simulink model "Simscape_Actuated_Robot"  (R2025b)
settings: Solver=ode45  StartTime=0.0  StopTime=20  RelTol=1e-3
InitFcn:
  | run("init.m");
values from neighbouring files (symbols this model uses):
  q0_guess = [pi/3; -pi/6; pi/3]    [init.m]
  q_init = [pi/6,-pi/3, 0,pi/6,-pi/3,0]    [init.m]
  Ts = 1e-3    (= 0.001)    [init.m]
undefined symbols (not defined in the file or in its folder): robot_params, X, Y, Z
libraries: sm_lib x48, nesl_utility x48
(part 2 of 3)

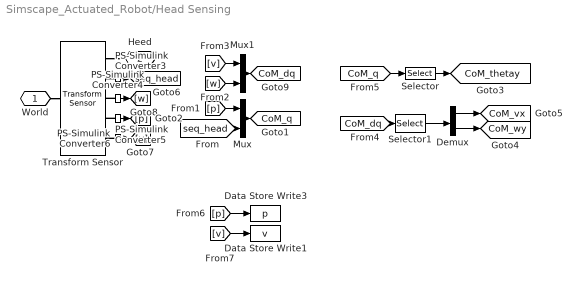
== system Simscape_Actuated_Robot/Head Sensing ==
  Data Store Write1 : DataStoreWrite  DataStoreName=v  DataStoreElements=v  EnableIndexing=on  NumberOfDimensions=2  IndexOptions=Index vector (dialog),Index vector (dialog)  Indices=[1 2 3],[2]  OutputSizes=1,1
  Data Store Write3 : DataStoreWrite  DataStoreName=p  DataStoreElements=p  EnableIndexing=on  NumberOfDimensions=2  IndexOptions=Index vector (dialog),Index vector (dialog)  Indices=[1 2 3],[1]  OutputSizes=1,1
  Demux : Demux  Outputs=2
  Mux : Mux  Inputs=2
  Mux1 : Mux  Inputs=2
  PS-Simulink Converter{3..6} (4 alike) : nesl_utility/PS-Simulink Converter  PhysicalDomain=network_engine_domain  SubClassName=ps_output  LeftPortType=input  RightPortType=output  PseudoPeriodic=off  Frequencies=[]  VectorFormat=inherit  Unit=inherit  AffineConversion=off
  Selector : Selector  InputPortWidth=6  IndexOptions=Index vector (dialog)  Indices=5  OutputSizes=1
  Selector1 : Selector  InputPortWidth=6  IndexOptions=Index vector (dialog)  Indices=[1 5]  OutputSizes=1
  Transform Sensor : sm_lib/Frames and Transforms/Transform Sensor  MeasurementFrame=World  RotationSequence=XYZ  SenseAngle=off  SenseAxis=off  SenseQ=off  SenseR=off  SenseRotationSequence=on  SenseOmegaX=off  SenseOmegaY=off  SenseOmegaZ=off  SenseOmega=on  SenseQDot=off  SenseRDot=off  SenseRotationSequenceDot=off  SenseAlphaX=off  SenseAlphaY=off  SenseAlphaZ=off  SenseAlpha=off  SenseQDDot=off  SenseRDDot=off  SenseX=off  SenseY=off  SenseZ=off  SenseXYZ=on  SenseRad=off  SenseAzim=off  SenseDist=off  SenseInc=off  SenseXDot=off  SenseYDot=off  SenseZDot=off  SenseXYZDot=on  SenseRadDot=off  SenseAzimDot=off  SenseDistDot=off  SenseIncDot=off  SenseXDDot=off  SenseYDDot=off  SenseZDDot=off  SenseXYZDDot=off  SenseRadDDot=off  SenseAzimDDot=off  SenseDistDDot=off  SenseIncDDot=off
  World : PMIOPort  Side=Right
  Heed : PMIOPort  Port=2  Side=Left
  tag scope: CoM_dq=global, CoM_q=global, CoM_thetay=global, CoM_vx=global, CoM_wy=global, seq_head=global
  wires:
  Selector/1 -> [CoM_thetay]
  PS-Simulink Converter5/1 -> [p]
  PS-Simulink Converter3/1 -> [seq_head]
  [p] -> Mux/1
  [seq_head] -> Mux/2
  PS-Simulink Converter6/1 -> [v]
  PS-Simulink Converter4/1 -> [w]
  Mux/1 -> [CoM_q]
  Mux1/1 -> [CoM_dq]
  [w] -> Mux1/2
  [v] -> Mux1/1
  [CoM_dq] -> Selector1/1
  Selector1/1 -> Demux/1
  Demux/1 -> [CoM_vx]
  Demux/2 -> [CoM_wy]
  [CoM_q] -> Selector/1
  [p] -> Data Store Write3/1
  [v] -> Data Store Write1/1
  connections:
  PS-Simulink Converter6/LConn1 -- Transform Sensor/RConn5
  PS-Simulink Converter5/LConn1 -- Transform Sensor/RConn4
  PS-Simulink Converter4/LConn1 -- Transform Sensor/RConn3
  Transform Sensor/RConn2 -- PS-Simulink Converter3/LConn1
  Transform Sensor/RConn1 -- Heed/RConn1
  World/RConn1 -- Transform Sensor/LConn1

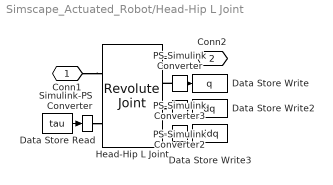
== system Simscape_Actuated_Robot/Head-Hip L Joint  ==
  Data Store Read : DataStoreRead  DataStoreName=tau  DataStoreElements=tau  EnableIndexing=on  IndexOptions=Index vector (dialog)  Indices=4  OutputSizes=1
  Data Store Write : DataStoreWrite  DataStoreName=q  DataStoreElements=q  EnableIndexing=on  IndexOptions=Index vector (dialog)  Indices=4  OutputSizes=1
  Data Store Write2 : DataStoreWrite  DataStoreName=dq  DataStoreElements=dq  EnableIndexing=on  IndexOptions=Index vector (dialog)  Indices=4  OutputSizes=1
  Data Store Write3 : DataStoreWrite  DataStoreName=ddq  DataStoreElements=ddq  EnableIndexing=on  IndexOptions=Index vector (dialog)  Indices=4  OutputSizes=1
  "Head-Hip L Joint " : sm_lib/Joints/Revolute Joint  JointMode=Normal  CompositeWrenchDir=FollowerOnBase  CompositeWrenchFrame=BaseFrame  SenseConstraintForce=off  SenseConstraintTorque=off  SenseTotalForce=off  SenseTotalTorque=off  PositionTargetSpecify=on  PositionTargetPriority=High  PositionTargetValue=q_init(4)  PositionTargetValueUnits=rad  VelocityTargetSpecify=off  VelocityTargetPriority=High  VelocityTargetValue=0  VelocityTargetValueUnits=rad/s  EquilibriumPosition=0  EquilibriumPositionUnits=rad  SpringStiffness=Motor_stiffness  SpringStiffnessUnits=N*m/deg  DampingCoefficient=Motor_damping  DampingCoefficientUnits=N*m/(deg/s)  LowerLimitSpecify=off  LowerLimitBound=-90  LowerLimitBoundUnits=deg  LowerLimitStiffness=1e4  LowerLimitStiffnessUnits=N*m/deg  LowerLimitDamping=10  LowerLimitDampingUnits=N*m/(deg/s)  LowerLimitTransitionRegionWidth=0.1  LowerLimitTransitionRegionWidthUnits=deg  UpperLimitSpecify=off  UpperLimitBound=90  UpperLimitBoundUnits=deg  UpperLimitStiffness=1e4  UpperLimitStiffnessUnits=N*m/deg  UpperLimitDamping=10  UpperLimitDampingUnits=N*m/(deg/s)  UpperLimitTransitionRegionWidth=0.1  UpperLimitTransitionRegionWidthUnits=deg  TorqueActuationMode=InputTorque  MotionActuationMode=ComputedMotion  SensePosition=on  SenseVelocity=on  SenseAcceleration=on  SenseTorqueForce=off  SenseLowerLimitTorqueForce=off  SenseUpperLimitTorqueForce=off
  PS-Simulink Converter : nesl_utility/PS-Simulink Converter  PhysicalDomain=network_engine_domain  SubClassName=ps_output  LeftPortType=input  RightPortType=output  PseudoPeriodic=off  Frequencies=[]  VectorFormat=1-D array  Unit=rad  AffineConversion=off
  PS-Simulink Converter2 : nesl_utility/PS-Simulink Converter  PhysicalDomain=network_engine_domain  SubClassName=ps_output  LeftPortType=input  RightPortType=output  PseudoPeriodic=off  Frequencies=[]  VectorFormat=1-D array  Unit=rad/s  AffineConversion=off
  PS-Simulink Converter3 : nesl_utility/PS-Simulink Converter  PhysicalDomain=network_engine_domain  SubClassName=ps_output  LeftPortType=input  RightPortType=output  PseudoPeriodic=off  Frequencies=[]  VectorFormat=inherit  Unit=inherit  AffineConversion=off
  Simulink-PS Converter : nesl_utility/Simulink-PS Converter  PhysicalDomain=network_engine_domain  SubClassName=ps_input  LeftPortType=input  RightPortType=output  PseudoPeriodic=off  Frequencies=[]  NoiseDistribution=none  NoiseParameters=[]  Unit=N*m  AffineConversion=off  FilteringAndDerivatives=provide  SimscapeFilterOrder=1  InputFilterTimeConstant=0.001  UdotUserProvided=0
  Conn1 : PMIOPort  Side=Left
  Conn2 : PMIOPort  Port=2  Side=Right
  wires:
  PS-Simulink Converter/1 -> Data Store Write/1
  PS-Simulink Converter2/1 -> Data Store Write2/1
  PS-Simulink Converter3/1 -> Data Store Write3/1
  Data Store Read/1 -> Simulink-PS Converter/1
  connections:
  Conn2/RConn1 -- "Head-Hip L Joint "/RConn1
  Conn1/RConn1 -- "Head-Hip L Joint "/LConn1
  PS-Simulink Converter/LConn1 -- "Head-Hip L Joint "/RConn2
  "Head-Hip L Joint "/RConn3 -- PS-Simulink Converter2/LConn1
  "Head-Hip L Joint "/RConn4 -- PS-Simulink Converter3/LConn1
  Simulink-PS Converter/RConn1 -- "Head-Hip L Joint "/LConn2

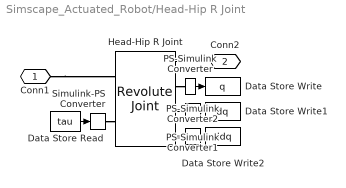
== system Simscape_Actuated_Robot/Head-Hip R Joint  ==
  Data Store Read : DataStoreRead  DataStoreName=tau  DataStoreElements=tau  EnableIndexing=on  IndexOptions=Index vector (dialog)  Indices=1  OutputSizes=1
  Data Store Write : DataStoreWrite  DataStoreName=q  DataStoreElements=q  EnableIndexing=on  IndexOptions=Index vector (dialog)  Indices=1  OutputSizes=1
  Data Store Write1 : DataStoreWrite  DataStoreName=dq  DataStoreElements=dq  EnableIndexing=on  IndexOptions=Index vector (dialog)  Indices=1  OutputSizes=1
  Data Store Write2 : DataStoreWrite  DataStoreName=ddq  DataStoreElements=ddq  EnableIndexing=on  IndexOptions=Index vector (dialog)  Indices=1  OutputSizes=1
  "Head-Hip R Joint " : sm_lib/Joints/Revolute Joint  JointMode=Normal  CompositeWrenchDir=FollowerOnBase  CompositeWrenchFrame=BaseFrame  SenseConstraintForce=off  SenseConstraintTorque=off  SenseTotalForce=off  SenseTotalTorque=off  PositionTargetSpecify=on  PositionTargetPriority=High  PositionTargetValue=q_init(1)  PositionTargetValueUnits=rad  VelocityTargetSpecify=off  VelocityTargetPriority=High  VelocityTargetValue=0  VelocityTargetValueUnits=deg/s  EquilibriumPosition=0  EquilibriumPositionUnits=rad  SpringStiffness=Motor_stiffness  SpringStiffnessUnits=N*m/deg  DampingCoefficient=Motor_damping  DampingCoefficientUnits=N*m/(deg/s)  LowerLimitSpecify=off  LowerLimitBound=-90  LowerLimitBoundUnits=deg  LowerLimitStiffness=1e4  LowerLimitStiffnessUnits=N*m/deg  LowerLimitDamping=10  LowerLimitDampingUnits=N*m/(deg/s)  LowerLimitTransitionRegionWidth=0.1  LowerLimitTransitionRegionWidthUnits=deg  UpperLimitSpecify=off  UpperLimitBound=90  UpperLimitBoundUnits=deg  UpperLimitStiffness=1e4  UpperLimitStiffnessUnits=N*m/deg  UpperLimitDamping=10  UpperLimitDampingUnits=N*m/(deg/s)  UpperLimitTransitionRegionWidth=0.1  UpperLimitTransitionRegionWidthUnits=deg  TorqueActuationMode=InputTorque  MotionActuationMode=ComputedMotion  SensePosition=on  SenseVelocity=on  SenseAcceleration=on  SenseTorqueForce=off  SenseLowerLimitTorqueForce=off  SenseUpperLimitTorqueForce=off
  PS-Simulink Converter : nesl_utility/PS-Simulink Converter  PhysicalDomain=network_engine_domain  SubClassName=ps_output  LeftPortType=input  RightPortType=output  PseudoPeriodic=off  Frequencies=[]  VectorFormat=1-D array  Unit=rad  AffineConversion=off
  PS-Simulink Converter1 : nesl_utility/PS-Simulink Converter  PhysicalDomain=network_engine_domain  SubClassName=ps_output  LeftPortType=input  RightPortType=output  PseudoPeriodic=off  Frequencies=[]  VectorFormat=1-D array  Unit=rad/s  AffineConversion=off
  PS-Simulink Converter2 : nesl_utility/PS-Simulink Converter  PhysicalDomain=network_engine_domain  SubClassName=ps_output  LeftPortType=input  RightPortType=output  PseudoPeriodic=off  Frequencies=[]  VectorFormat=1-D array  Unit=inherit  AffineConversion=off
  Simulink-PS Converter : nesl_utility/Simulink-PS Converter  PhysicalDomain=network_engine_domain  SubClassName=ps_input  LeftPortType=input  RightPortType=output  PseudoPeriodic=off  Frequencies=[]  NoiseDistribution=none  NoiseParameters=[]  Unit=N*m  AffineConversion=off  FilteringAndDerivatives=provide  SimscapeFilterOrder=1  InputFilterTimeConstant=0.001  UdotUserProvided=0
  Conn1 : PMIOPort  Side=Left
  Conn2 : PMIOPort  Port=2  Side=Right
  wires:
  PS-Simulink Converter/1 -> Data Store Write/1
  PS-Simulink Converter1/1 -> Data Store Write1/1
  PS-Simulink Converter2/1 -> Data Store Write2/1
  Data Store Read/1 -> Simulink-PS Converter/1
  connections:
  PS-Simulink Converter1/LConn1 -- "Head-Hip R Joint "/RConn3
  Conn2/RConn1 -- "Head-Hip R Joint "/RConn1
  "Head-Hip R Joint "/RConn2 -- PS-Simulink Converter/LConn1
  Conn1/RConn1 -- "Head-Hip R Joint "/LConn1
  PS-Simulink Converter2/LConn1 -- "Head-Hip R Joint "/RConn4
  Simulink-PS Converter/RConn1 -- "Head-Hip R Joint "/LConn2

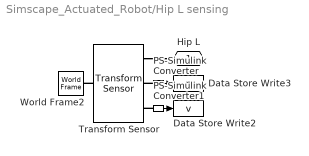
== system Simscape_Actuated_Robot/Hip L sensing ==
  Data Store Write2 : DataStoreWrite  DataStoreName=v  DataStoreElements=v  EnableIndexing=on  NumberOfDimensions=2  IndexOptions=Index vector (dialog),Index vector (dialog)  Indices=[1 2 3],[4]  OutputSizes=1,1
  Data Store Write3 : DataStoreWrite  DataStoreName=p  DataStoreElements=p  EnableIndexing=on  NumberOfDimensions=2  IndexOptions=Index vector (dialog),Index vector (dialog)  Indices=[1 2 3],[4]  OutputSizes=1,1
  PS-Simulink Converter : nesl_utility/PS-Simulink Converter  PhysicalDomain=network_engine_domain  SubClassName=ps_output  LeftPortType=input  RightPortType=output  PseudoPeriodic=off  Frequencies=[]  VectorFormat=inherit  Unit=inherit  AffineConversion=off
  PS-Simulink Converter1 : nesl_utility/PS-Simulink Converter  PhysicalDomain=network_engine_domain  SubClassName=ps_output  LeftPortType=input  RightPortType=output  PseudoPeriodic=off  Frequencies=[]  VectorFormat=inherit  Unit=inherit  AffineConversion=off
  Transform Sensor : sm_lib/Frames and Transforms/Transform Sensor  MeasurementFrame=World  RotationSequence=XYX  SenseAngle=off  SenseAxis=off  SenseQ=off  SenseR=off  SenseRotationSequence=off  SenseOmegaX=off  SenseOmegaY=off  SenseOmegaZ=off  SenseOmega=off  SenseQDot=off  SenseRDot=off  SenseRotationSequenceDot=off  SenseAlphaX=off  SenseAlphaY=off  SenseAlphaZ=off  SenseAlpha=off  SenseQDDot=off  SenseRDDot=off  SenseX=off  SenseY=off  SenseZ=off  SenseXYZ=on  SenseRad=off  SenseAzim=off  SenseDist=off  SenseInc=off  SenseXDot=off  SenseYDot=off  SenseZDot=off  SenseXYZDot=on  SenseRadDot=off  SenseAzimDot=off  SenseDistDot=off  SenseIncDot=off  SenseXDDot=off  SenseYDDot=off  SenseZDDot=off  SenseXYZDDot=off  SenseRadDDot=off  SenseAzimDDot=off  SenseDistDDot=off  SenseIncDDot=off
  World Frame2 : sm_lib/Frames and Transforms/World Frame
  Hip L : PMIOPort  Side=Right
  wires:
  PS-Simulink Converter/1 -> Data Store Write3/1
  PS-Simulink Converter1/1 -> Data Store Write2/1
  connections:
  PS-Simulink Converter/LConn1 -- Transform Sensor/RConn2
  Transform Sensor/RConn1 -- Hip L/RConn1
  Transform Sensor/LConn1 -- World Frame2/RConn1
  PS-Simulink Converter1/LConn1 -- Transform Sensor/RConn3

== system Simscape_Actuated_Robot/Hip R sensing ==
  Data Store Write1 : DataStoreWrite  DataStoreName=v  DataStoreElements=v  EnableIndexing=on  NumberOfDimensions=2  IndexOptions=Index vector (dialog),Index vector (dialog)  Indices=[1 2 3],[2]  OutputSizes=1,1
  Data Store Write3 : DataStoreWrite  DataStoreName=p  DataStoreElements=p  EnableIndexing=on  NumberOfDimensions=2  IndexOptions=Index vector (dialog),Index vector (dialog)  Indices=[1 2 3],[2]  OutputSizes=1,1
  PS-Simulink Converter : nesl_utility/PS-Simulink Converter  PhysicalDomain=network_engine_domain  SubClassName=ps_output  LeftPortType=input  RightPortType=output  PseudoPeriodic=off  Frequencies=[]  VectorFormat=inherit  Unit=inherit  AffineConversion=off
  PS-Simulink Converter1 : nesl_utility/PS-Simulink Converter  PhysicalDomain=network_engine_domain  SubClassName=ps_output  LeftPortType=input  RightPortType=output  PseudoPeriodic=off  Frequencies=[]  VectorFormat=inherit  Unit=inherit  AffineConversion=off
  Transform Sensor : sm_lib/Frames and Transforms/Transform Sensor  MeasurementFrame=World  RotationSequence=XYX  SenseAngle=off  SenseAxis=off  SenseQ=off  SenseR=off  SenseRotationSequence=off  SenseOmegaX=off  SenseOmegaY=off  SenseOmegaZ=off  SenseOmega=off  SenseQDot=off  SenseRDot=off  SenseRotationSequenceDot=off  SenseAlphaX=off  SenseAlphaY=off  SenseAlphaZ=off  SenseAlpha=off  SenseQDDot=off  SenseRDDot=off  SenseX=off  SenseY=off  SenseZ=off  SenseXYZ=on  SenseRad=off  SenseAzim=off  SenseDist=off  SenseInc=off  SenseXDot=off  SenseYDot=off  SenseZDot=off  SenseXYZDot=on  SenseRadDot=off  SenseAzimDot=off  SenseDistDot=off  SenseIncDot=off  SenseXDDot=off  SenseYDDot=off  SenseZDDot=off  SenseXYZDDot=off  SenseRadDDot=off  SenseAzimDDot=off  SenseDistDDot=off  SenseIncDDot=off
  World Frame2 : sm_lib/Frames and Transforms/World Frame
  Hip R : PMIOPort  Side=Right
  wires:
  PS-Simulink Converter/1 -> Data Store Write3/1
  PS-Simulink Converter1/1 -> Data Store Write1/1
  connections:
  Transform Sensor/LConn1 -- World Frame2/RConn1
  Transform Sensor/RConn1 -- Hip R/RConn1
  PS-Simulink Converter/LConn1 -- Transform Sensor/RConn2
  PS-Simulink Converter1/LConn1 -- Transform Sensor/RConn3

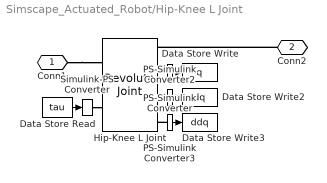
== system Simscape_Actuated_Robot/Hip-Knee L Joint ==
  Data Store Read : DataStoreRead  DataStoreName=tau  DataStoreElements=tau  EnableIndexing=on  IndexOptions=Index vector (dialog)  Indices=5  OutputSizes=1
  Data Store Write : DataStoreWrite  DataStoreName=q  DataStoreElements=q  EnableIndexing=on  IndexOptions=Index vector (dialog)  Indices=5  OutputSizes=1
  Data Store Write2 : DataStoreWrite  DataStoreName=dq  DataStoreElements=dq  EnableIndexing=on  IndexOptions=Index vector (dialog)  Indices=5  OutputSizes=1
  Data Store Write3 : DataStoreWrite  DataStoreName=ddq  DataStoreElements=ddq  EnableIndexing=on  IndexOptions=Index vector (dialog)  Indices=5  OutputSizes=1
  Hip-Knee L Joint : sm_lib/Joints/Revolute Joint  JointMode=Normal  CompositeWrenchDir=FollowerOnBase  CompositeWrenchFrame=BaseFrame  SenseConstraintForce=off  SenseConstraintTorque=off  SenseTotalForce=off  SenseTotalTorque=off  PositionTargetSpecify=on  PositionTargetPriority=High  PositionTargetValue=q_init(5)  PositionTargetValueUnits=rad  VelocityTargetSpecify=off  VelocityTargetPriority=High  VelocityTargetValue=0  VelocityTargetValueUnits=deg/s  EquilibriumPosition=0  EquilibriumPositionUnits=deg  SpringStiffness=Motor_stiffness  SpringStiffnessUnits=N*m/deg  DampingCoefficient=Motor_damping  DampingCoefficientUnits=N*m/(deg/s)  LowerLimitSpecify=off  LowerLimitBound=-90  LowerLimitBoundUnits=deg  LowerLimitStiffness=1e4  LowerLimitStiffnessUnits=N*m/deg  LowerLimitDamping=10  LowerLimitDampingUnits=N*m/(deg/s)  LowerLimitTransitionRegionWidth=0.1  LowerLimitTransitionRegionWidthUnits=deg  UpperLimitSpecify=off  UpperLimitBound=90  UpperLimitBoundUnits=deg  UpperLimitStiffness=1e4  UpperLimitStiffnessUnits=N*m/deg  UpperLimitDamping=10  UpperLimitDampingUnits=N*m/(deg/s)  UpperLimitTransitionRegionWidth=0.1  UpperLimitTransitionRegionWidthUnits=deg  TorqueActuationMode=InputTorque  MotionActuationMode=ComputedMotion  SensePosition=on  SenseVelocity=on  SenseAcceleration=on  SenseTorqueForce=off  SenseLowerLimitTorqueForce=off  SenseUpperLimitTorqueForce=off
  PS-Simulink Converter : nesl_utility/PS-Simulink Converter  PhysicalDomain=network_engine_domain  SubClassName=ps_output  LeftPortType=input  RightPortType=output  PseudoPeriodic=off  Frequencies=[]  VectorFormat=1-D array  Unit=rad  AffineConversion=off
  PS-Simulink Converter2 : nesl_utility/PS-Simulink Converter  PhysicalDomain=network_engine_domain  SubClassName=ps_output  LeftPortType=input  RightPortType=output  PseudoPeriodic=off  Frequencies=[]  VectorFormat=1-D array  Unit=rad/s  AffineConversion=off
  PS-Simulink Converter3 : nesl_utility/PS-Simulink Converter  PhysicalDomain=network_engine_domain  SubClassName=ps_output  LeftPortType=input  RightPortType=output  PseudoPeriodic=off  Frequencies=[]  VectorFormat=inherit  Unit=inherit  AffineConversion=off
  Simulink-PS Converter : nesl_utility/Simulink-PS Converter  PhysicalDomain=network_engine_domain  SubClassName=ps_input  LeftPortType=input  RightPortType=output  PseudoPeriodic=off  Frequencies=[]  NoiseDistribution=none  NoiseParameters=[]  Unit=N*m  AffineConversion=off  FilteringAndDerivatives=provide  SimscapeFilterOrder=1  InputFilterTimeConstant=0.001  UdotUserProvided=0
  Conn1 : PMIOPort  Side=Left
  Conn2 : PMIOPort  Port=2  Side=Right
  wires:
  PS-Simulink Converter/1 -> Data Store Write/1
  PS-Simulink Converter3/1 -> Data Store Write3/1
  PS-Simulink Converter2/1 -> Data Store Write2/1
  Data Store Read/1 -> Simulink-PS Converter/1
  connections:
  Conn2/RConn1 -- Hip-Knee L Joint/RConn1
  Conn1/RConn1 -- Hip-Knee L Joint/LConn1
  PS-Simulink Converter/LConn1 -- Hip-Knee L Joint/RConn2
  PS-Simulink Converter3/LConn1 -- Hip-Knee L Joint/RConn4
  PS-Simulink Converter2/LConn1 -- Hip-Knee L Joint/RConn3
  Simulink-PS Converter/RConn1 -- Hip-Knee L Joint/LConn2

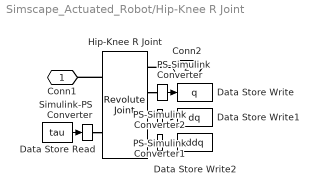
== system Simscape_Actuated_Robot/Hip-Knee R Joint ==
  Data Store Read : DataStoreRead  DataStoreName=tau  DataStoreElements=tau  EnableIndexing=on  IndexOptions=Index vector (dialog)  Indices=2  OutputSizes=1
  Data Store Write : DataStoreWrite  DataStoreName=q  DataStoreElements=q  EnableIndexing=on  IndexOptions=Index vector (dialog)  Indices=2  OutputSizes=1
  Data Store Write1 : DataStoreWrite  DataStoreName=dq  DataStoreElements=dq  EnableIndexing=on  IndexOptions=Index vector (dialog)  Indices=2  OutputSizes=1
  Data Store Write2 : DataStoreWrite  DataStoreName=ddq  DataStoreElements=ddq  EnableIndexing=on  IndexOptions=Index vector (dialog)  Indices=2  OutputSizes=1
  Hip-Knee R Joint : sm_lib/Joints/Revolute Joint  JointMode=Normal  CompositeWrenchDir=FollowerOnBase  CompositeWrenchFrame=BaseFrame  SenseConstraintForce=off  SenseConstraintTorque=off  SenseTotalForce=off  SenseTotalTorque=off  PositionTargetSpecify=on  PositionTargetPriority=High  PositionTargetValue=q_init(2)  PositionTargetValueUnits=rad  VelocityTargetSpecify=off  VelocityTargetPriority=High  VelocityTargetValue=0  VelocityTargetValueUnits=deg/s  EquilibriumPosition=0  EquilibriumPositionUnits=deg  SpringStiffness=Motor_stiffness  SpringStiffnessUnits=N*m/deg  DampingCoefficient=Motor_damping  DampingCoefficientUnits=N*m/(deg/s)  LowerLimitSpecify=off  LowerLimitBound=-90  LowerLimitBoundUnits=deg  LowerLimitStiffness=1e4  LowerLimitStiffnessUnits=N*m/deg  LowerLimitDamping=10  LowerLimitDampingUnits=N*m/(deg/s)  LowerLimitTransitionRegionWidth=0.1  LowerLimitTransitionRegionWidthUnits=deg  UpperLimitSpecify=off  UpperLimitBound=90  UpperLimitBoundUnits=deg  UpperLimitStiffness=1e4  UpperLimitStiffnessUnits=N*m/deg  UpperLimitDamping=10  UpperLimitDampingUnits=N*m/(deg/s)  UpperLimitTransitionRegionWidth=0.1  UpperLimitTransitionRegionWidthUnits=deg  TorqueActuationMode=InputTorque  MotionActuationMode=ComputedMotion  SensePosition=on  SenseVelocity=on  SenseAcceleration=on  SenseTorqueForce=off  SenseLowerLimitTorqueForce=off  SenseUpperLimitTorqueForce=off
  PS-Simulink Converter : nesl_utility/PS-Simulink Converter  PhysicalDomain=network_engine_domain  SubClassName=ps_output  LeftPortType=input  RightPortType=output  PseudoPeriodic=off  Frequencies=[]  VectorFormat=1-D array  Unit=rad  AffineConversion=off
  PS-Simulink Converter1 : nesl_utility/PS-Simulink Converter  PhysicalDomain=network_engine_domain  SubClassName=ps_output  LeftPortType=input  RightPortType=output  PseudoPeriodic=off  Frequencies=[]  VectorFormat=1-D array  Unit=rad/s  AffineConversion=off
  PS-Simulink Converter2 : nesl_utility/PS-Simulink Converter  PhysicalDomain=network_engine_domain  SubClassName=ps_output  LeftPortType=input  RightPortType=output  PseudoPeriodic=off  Frequencies=[]  VectorFormat=inherit  Unit=inherit  AffineConversion=off
  Simulink-PS Converter : nesl_utility/Simulink-PS Converter  PhysicalDomain=network_engine_domain  SubClassName=ps_input  LeftPortType=input  RightPortType=output  PseudoPeriodic=off  Frequencies=[]  NoiseDistribution=none  NoiseParameters=[]  Unit=N*m  AffineConversion=off  FilteringAndDerivatives=provide  SimscapeFilterOrder=1  InputFilterTimeConstant=0.001  UdotUserProvided=0
  Conn1 : PMIOPort  Side=Left
  Conn2 : PMIOPort  Port=2  Side=Right
  wires:
  PS-Simulink Converter/1 -> Data Store Write/1
  PS-Simulink Converter2/1 -> Data Store Write2/1
  PS-Simulink Converter1/1 -> Data Store Write1/1
  Data Store Read/1 -> Simulink-PS Converter/1
  connections:
  Conn2/RConn1 -- Hip-Knee R Joint/RConn1
  Hip-Knee R Joint/LConn1 -- Conn1/RConn1
  Hip-Knee R Joint/RConn2 -- PS-Simulink Converter/LConn1
  PS-Simulink Converter1/LConn1 -- Hip-Knee R Joint/RConn3
  PS-Simulink Converter2/LConn1 -- Hip-Knee R Joint/RConn4
  Simulink-PS Converter/RConn1 -- Hip-Knee R Joint/LConn2

== system Simscape_Actuated_Robot/Knee L sensing ==
  Data Store Write1 : DataStoreWrite  DataStoreName=v  DataStoreElements=v  EnableIndexing=on  NumberOfDimensions=2  IndexOptions=Index vector (dialog),Index vector (dialog)  Indices=[1 2 3],[5]  OutputSizes=1,1
  Data Store Write3 : DataStoreWrite  DataStoreName=p  DataStoreElements=p  EnableIndexing=on  NumberOfDimensions=2  IndexOptions=Index vector (dialog),Index vector (dialog)  Indices=[1 2 3],[5]  OutputSizes=1,1
  PS-Simulink Converter : nesl_utility/PS-Simulink Converter  PhysicalDomain=network_engine_domain  SubClassName=ps_output  LeftPortType=input  RightPortType=output  PseudoPeriodic=off  Frequencies=[]  VectorFormat=inherit  Unit=inherit  AffineConversion=off
  PS-Simulink Converter1 : nesl_utility/PS-Simulink Converter  PhysicalDomain=network_engine_domain  SubClassName=ps_output  LeftPortType=input  RightPortType=output  PseudoPeriodic=off  Frequencies=[]  VectorFormat=inherit  Unit=inherit  AffineConversion=off
  Transform Sensor : sm_lib/Frames and Transforms/Transform Sensor  MeasurementFrame=World  RotationSequence=XYX  SenseAngle=off  SenseAxis=off  SenseQ=off  SenseR=off  SenseRotationSequence=off  SenseOmegaX=off  SenseOmegaY=off  SenseOmegaZ=off  SenseOmega=off  SenseQDot=off  SenseRDot=off  SenseRotationSequenceDot=off  SenseAlphaX=off  SenseAlphaY=off  SenseAlphaZ=off  SenseAlpha=off  SenseQDDot=off  SenseRDDot=off  SenseX=off  SenseY=off  SenseZ=off  SenseXYZ=on  SenseRad=off  SenseAzim=off  SenseDist=off  SenseInc=off  SenseXDot=off  SenseYDot=off  SenseZDot=off  SenseXYZDot=on  SenseRadDot=off  SenseAzimDot=off  SenseDistDot=off  SenseIncDot=off  SenseXDDot=off  SenseYDDot=off  SenseZDDot=off  SenseXYZDDot=off  SenseRadDDot=off  SenseAzimDDot=off  SenseDistDDot=off  SenseIncDDot=off
  World Frame2 : sm_lib/Frames and Transforms/World Frame
  Knee L : PMIOPort  Side=Right
  wires:
  PS-Simulink Converter/1 -> Data Store Write3/1
  PS-Simulink Converter1/1 -> Data Store Write1/1
  connections:
  Transform Sensor/LConn1 -- World Frame2/RConn1
  Transform Sensor/RConn1 -- Knee L/RConn1
  PS-Simulink Converter/LConn1 -- Transform Sensor/RConn2
  PS-Simulink Converter1/LConn1 -- Transform Sensor/RConn3

== system Simscape_Actuated_Robot/Knee R sensing ==
  Data Store Write1 : DataStoreWrite  DataStoreName=v  DataStoreElements=v  EnableIndexing=on  NumberOfDimensions=2  IndexOptions=Index vector (dialog),Index vector (dialog)  Indices=[1 2 3],[3]  OutputSizes=1,1
  Data Store Write3 : DataStoreWrite  DataStoreName=p  DataStoreElements=p  EnableIndexing=on  NumberOfDimensions=2  IndexOptions=Index vector (dialog),Index vector (dialog)  Indices=[1 2 3],[3]  OutputSizes=1,1
  PS-Simulink Converter : nesl_utility/PS-Simulink Converter  PhysicalDomain=network_engine_domain  SubClassName=ps_output  LeftPortType=input  RightPortType=output  PseudoPeriodic=off  Frequencies=[]  VectorFormat=inherit  Unit=inherit  AffineConversion=off
  PS-Simulink Converter1 : nesl_utility/PS-Simulink Converter  PhysicalDomain=network_engine_domain  SubClassName=ps_output  LeftPortType=input  RightPortType=output  PseudoPeriodic=off  Frequencies=[]  VectorFormat=inherit  Unit=inherit  AffineConversion=off
  Transform Sensor : sm_lib/Frames and Transforms/Transform Sensor  MeasurementFrame=World  RotationSequence=XYX  SenseAngle=off  SenseAxis=off  SenseQ=off  SenseR=off  SenseRotationSequence=off  SenseOmegaX=off  SenseOmegaY=off  SenseOmegaZ=off  SenseOmega=off  SenseQDot=off  SenseRDot=off  SenseRotationSequenceDot=off  SenseAlphaX=off  SenseAlphaY=off  SenseAlphaZ=off  SenseAlpha=off  SenseQDDot=off  SenseRDDot=off  SenseX=off  SenseY=off  SenseZ=off  SenseXYZ=on  SenseRad=off  SenseAzim=off  SenseDist=off  SenseInc=off  SenseXDot=off  SenseYDot=off  SenseZDot=off  SenseXYZDot=on  SenseRadDot=off  SenseAzimDot=off  SenseDistDot=off  SenseIncDot=off  SenseXDDot=off  SenseYDDot=off  SenseZDDot=off  SenseXYZDDot=off  SenseRadDDot=off  SenseAzimDDot=off  SenseDistDDot=off  SenseIncDDot=off
  World Frame2 : sm_lib/Frames and Transforms/World Frame
  Knee R : PMIOPort  Side=Right
  wires:
  PS-Simulink Converter/1 -> Data Store Write3/1
  PS-Simulink Converter1/1 -> Data Store Write1/1
  connections:
  PS-Simulink Converter/LConn1 -- Transform Sensor/RConn2
  Transform Sensor/RConn1 -- Knee R/RConn1
  Transform Sensor/LConn1 -- World Frame2/RConn1
  Transform Sensor/RConn3 -- PS-Simulink Converter1/LConn1

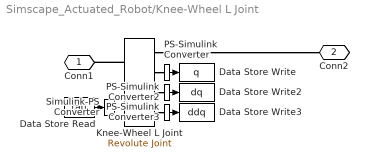
== system Simscape_Actuated_Robot/Knee-Wheel L Joint ==
  Data Store Read : DataStoreRead  DataStoreName=tau  DataStoreElements=tau  EnableIndexing=on  IndexOptions=Index vector (dialog)  Indices=6  OutputSizes=1
  Data Store Write : DataStoreWrite  DataStoreName=q  DataStoreElements=q  EnableIndexing=on  IndexOptions=Index vector (dialog)  Indices=6  OutputSizes=1
  Data Store Write2 : DataStoreWrite  DataStoreName=dq  DataStoreElements=dq  EnableIndexing=on  IndexOptions=Index vector (dialog)  Indices=6  OutputSizes=1
  Data Store Write3 : DataStoreWrite  DataStoreName=ddq  DataStoreElements=ddq  EnableIndexing=on  IndexOptions=Index vector (dialog)  Indices=6  OutputSizes=1
  Knee-Wheel L Joint : sm_lib/Joints/Revolute Joint  JointMode=Normal  CompositeWrenchDir=FollowerOnBase  CompositeWrenchFrame=BaseFrame  SenseConstraintForce=off  SenseConstraintTorque=off  SenseTotalForce=off  SenseTotalTorque=off  PositionTargetSpecify=on  PositionTargetPriority=High  PositionTargetValue=q_init(6)  PositionTargetValueUnits=rad  VelocityTargetSpecify=off  VelocityTargetPriority=High  VelocityTargetValue=0  VelocityTargetValueUnits=rad/s  EquilibriumPosition=0  EquilibriumPositionUnits=deg  SpringStiffness=Motor_stiffness  SpringStiffnessUnits=N*m/deg  DampingCoefficient=Motor_damping  DampingCoefficientUnits=N*m/(deg/s)  LowerLimitSpecify=off  LowerLimitBound=-90  LowerLimitBoundUnits=deg  LowerLimitStiffness=1e4  LowerLimitStiffnessUnits=N*m/deg  LowerLimitDamping=10  LowerLimitDampingUnits=N*m/(deg/s)  LowerLimitTransitionRegionWidth=0.1  LowerLimitTransitionRegionWidthUnits=deg  UpperLimitSpecify=off  UpperLimitBound=90  UpperLimitBoundUnits=deg  UpperLimitStiffness=1e4  UpperLimitStiffnessUnits=N*m/deg  UpperLimitDamping=10  UpperLimitDampingUnits=N*m/(deg/s)  UpperLimitTransitionRegionWidth=0.1  UpperLimitTransitionRegionWidthUnits=deg  TorqueActuationMode=InputTorque  MotionActuationMode=ComputedMotion  SensePosition=on  SenseVelocity=on  SenseAcceleration=on  SenseTorqueForce=off  SenseLowerLimitTorqueForce=off  SenseUpperLimitTorqueForce=off
  PS-Simulink Converter : nesl_utility/PS-Simulink Converter  PhysicalDomain=network_engine_domain  SubClassName=ps_output  LeftPortType=input  RightPortType=output  PseudoPeriodic=off  Frequencies=[]  VectorFormat=1-D array  Unit=rad  AffineConversion=off
  PS-Simulink Converter2 : nesl_utility/PS-Simulink Converter  PhysicalDomain=network_engine_domain  SubClassName=ps_output  LeftPortType=input  RightPortType=output  PseudoPeriodic=off  Frequencies=[]  VectorFormat=1-D array  Unit=rad/s  AffineConversion=off
  PS-Simulink Converter3 : nesl_utility/PS-Simulink Converter  PhysicalDomain=network_engine_domain  SubClassName=ps_output  LeftPortType=input  RightPortType=output  PseudoPeriodic=off  Frequencies=[]  VectorFormat=inherit  Unit=inherit  AffineConversion=off
  Simulink-PS Converter : nesl_utility/Simulink-PS Converter  PhysicalDomain=network_engine_domain  SubClassName=ps_input  LeftPortType=input  RightPortType=output  PseudoPeriodic=off  Frequencies=[]  NoiseDistribution=none  NoiseParameters=[]  Unit=N*m  AffineConversion=off  FilteringAndDerivatives=provide  SimscapeFilterOrder=1  InputFilterTimeConstant=0.001  UdotUserProvided=0
  Conn1 : PMIOPort  Side=Left
  Conn2 : PMIOPort  Port=2  Side=Right
  wires:
  PS-Simulink Converter3/1 -> Data Store Write3/1
  PS-Simulink Converter2/1 -> Data Store Write2/1
  PS-Simulink Converter/1 -> Data Store Write/1
  Data Store Read/1 -> Simulink-PS Converter/1
  connections:
  Knee-Wheel L Joint/RConn1 -- Conn2/RConn1
  Knee-Wheel L Joint/LConn1 -- Conn1/RConn1
  Knee-Wheel L Joint/RConn2 -- PS-Simulink Converter/LConn1
  Knee-Wheel L Joint/RConn3 -- PS-Simulink Converter2/LConn1
  Knee-Wheel L Joint/RConn4 -- PS-Simulink Converter3/LConn1
  Simulink-PS Converter/RConn1 -- Knee-Wheel L Joint/LConn2

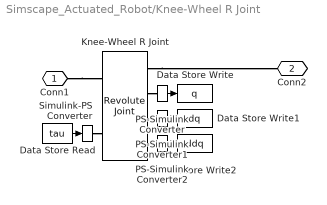
== system Simscape_Actuated_Robot/Knee-Wheel R Joint ==
  Data Store Read : DataStoreRead  DataStoreName=tau  DataStoreElements=tau  EnableIndexing=on  IndexOptions=Index vector (dialog)  Indices=3  OutputSizes=1
  Data Store Write : DataStoreWrite  DataStoreName=q  DataStoreElements=q  EnableIndexing=on  IndexOptions=Index vector (dialog)  Indices=3  OutputSizes=1
  Data Store Write1 : DataStoreWrite  DataStoreName=dq  DataStoreElements=dq  EnableIndexing=on  IndexOptions=Index vector (dialog)  Indices=3  OutputSizes=1
  Data Store Write2 : DataStoreWrite  DataStoreName=ddq  DataStoreElements=ddq  EnableIndexing=on  IndexOptions=Index vector (dialog)  Indices=3  OutputSizes=1
  Knee-Wheel R Joint : sm_lib/Joints/Revolute Joint  JointMode=Normal  CompositeWrenchDir=FollowerOnBase  CompositeWrenchFrame=BaseFrame  SenseConstraintForce=off  SenseConstraintTorque=off  SenseTotalForce=off  SenseTotalTorque=off  PositionTargetSpecify=on  PositionTargetPriority=High  PositionTargetValue=q_init(3)  PositionTargetValueUnits=deg  VelocityTargetSpecify=off  VelocityTargetPriority=High  VelocityTargetValue=q_init(3)  VelocityTargetValueUnits=rad/s  EquilibriumPosition=0  EquilibriumPositionUnits=deg  SpringStiffness=Motor_stiffness  SpringStiffnessUnits=N*m/deg  DampingCoefficient=Motor_damping  DampingCoefficientUnits=N*m/(deg/s)  LowerLimitSpecify=off  LowerLimitBound=-90  LowerLimitBoundUnits=deg  LowerLimitStiffness=1e4  LowerLimitStiffnessUnits=N*m/deg  LowerLimitDamping=10  LowerLimitDampingUnits=N*m/(deg/s)  LowerLimitTransitionRegionWidth=0.1  LowerLimitTransitionRegionWidthUnits=deg  UpperLimitSpecify=off  UpperLimitBound=90  UpperLimitBoundUnits=deg  UpperLimitStiffness=1e4  UpperLimitStiffnessUnits=N*m/deg  UpperLimitDamping=10  UpperLimitDampingUnits=N*m/(deg/s)  UpperLimitTransitionRegionWidth=0.1  UpperLimitTransitionRegionWidthUnits=deg  TorqueActuationMode=InputTorque  MotionActuationMode=ComputedMotion  SensePosition=on  SenseVelocity=on  SenseAcceleration=on  SenseTorqueForce=off  SenseLowerLimitTorqueForce=off  SenseUpperLimitTorqueForce=off
  PS-Simulink Converter : nesl_utility/PS-Simulink Converter  PhysicalDomain=network_engine_domain  SubClassName=ps_output  LeftPortType=input  RightPortType=output  PseudoPeriodic=off  Frequencies=[]  VectorFormat=1-D array  Unit=rad  AffineConversion=off
  PS-Simulink Converter1 : nesl_utility/PS-Simulink Converter  PhysicalDomain=network_engine_domain  SubClassName=ps_output  LeftPortType=input  RightPortType=output  PseudoPeriodic=off  Frequencies=[]  VectorFormat=1-D array  Unit=rad/s  AffineConversion=off
  PS-Simulink Converter2 : nesl_utility/PS-Simulink Converter  PhysicalDomain=network_engine_domain  SubClassName=ps_output  LeftPortType=input  RightPortType=output  PseudoPeriodic=off  Frequencies=[]  VectorFormat=inherit  Unit=inherit  AffineConversion=off
  Simulink-PS Converter : nesl_utility/Simulink-PS Converter  PhysicalDomain=network_engine_domain  SubClassName=ps_input  LeftPortType=input  RightPortType=output  PseudoPeriodic=off  Frequencies=[]  NoiseDistribution=none  NoiseParameters=[]  Unit=N*m  AffineConversion=off  FilteringAndDerivatives=provide  SimscapeFilterOrder=1  InputFilterTimeConstant=0.001  UdotUserProvided=0
  Conn1 : PMIOPort  Side=Left
  Conn2 : PMIOPort  Port=2  Side=Right
  wires:
  PS-Simulink Converter/1 -> Data Store Write/1
  PS-Simulink Converter1/1 -> Data Store Write1/1
  PS-Simulink Converter2/1 -> Data Store Write2/1
  Data Store Read/1 -> Simulink-PS Converter/1
  connections:
  Conn1/RConn1 -- Knee-Wheel R Joint/LConn1
  Knee-Wheel R Joint/RConn1 -- Conn2/RConn1
  Knee-Wheel R Joint/RConn2 -- PS-Simulink Converter/LConn1
  Knee-Wheel R Joint/RConn3 -- PS-Simulink Converter1/LConn1
  Knee-Wheel R Joint/RConn4 -- PS-Simulink Converter2/LConn1
  Simulink-PS Converter/RConn1 -- Knee-Wheel R Joint/LConn2

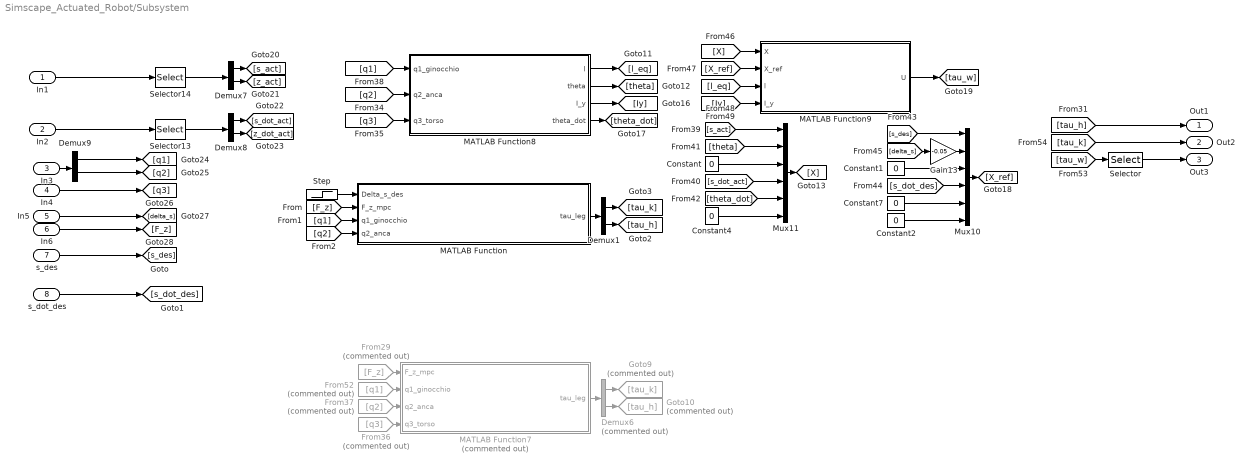
== system Simscape_Actuated_Robot/Subsystem ==
  In1 : Inport
  In2 : Inport  Port=2
  In3 : Inport  Port=3
  In4 : Inport  Port=4
  In5 : Inport  Port=5
  In6 : Inport  Port=6
  s_des : Inport  Port=7
  s_dot_des : Inport  Port=8
  Constant{,1..2,4,7} (5 alike) : Constant  Value=0
  Demux{1,7..9} (4 alike) : Demux  Outputs=2
  Demux6 : Demux  Commented=on  Outputs=2
  From29 : From  Commented=on  GotoTag=F_z
  From36 : From  Commented=on  GotoTag=q3
  From37 : From  Commented=on  GotoTag=q2
  From52 : From  Commented=on  GotoTag=q1
  Gain13 : Gain  Gain=-0.05
  Goto10 : Goto  Commented=on  GotoTag=tau_h
  Goto9 : Goto  Commented=on  GotoTag=tau_k
  MATLAB Function : MATLAB Function  TreatAsAtomicUnit=on
  MATLAB Function7 : MATLAB Function  Commented=on  TreatAsAtomicUnit=on
  MATLAB Function8 : MATLAB Function  TreatAsAtomicUnit=on
  MATLAB Function9 : MATLAB Function  TreatAsAtomicUnit=on
  Mux10 : Mux  Inputs=6
  Mux11 : Mux  Inputs=6
  Selector : Selector  InputPortWidth=2  IndexOptions=Index vector (dialog)  Indices=[1]  OutputSizes=1
  Selector13 : Selector  InputPortWidth=3  IndexOptions=Index vector (dialog)  Indices=[1 3]  OutputSizes=1
  Selector14 : Selector  InputPortWidth=3  IndexOptions=Index vector (dialog)  Indices=[1 3]  OutputSizes=1
  Step : Step  Time=2  After=0.05  SampleTime=0
  Out1 : Outport
  Out2 : Outport  Port=2
  Out3 : Outport  Port=3
  wires:
  Demux7/2 -> [z_act]
  From29/1 -> MATLAB Function7/1(F_z_mpc)
  [s_dot_des] -> Mux10/4
  [tau_h] -> Out1/1
  [q1] -> MATLAB Function8/1(q1_ginocchio)
  [q3] -> MATLAB Function8/3(q3_torso)
  From36/1 -> MATLAB Function7/4(q3_torso)
  Demux8/2 -> [z_dot_act]
  From37/1 -> MATLAB Function7/3(q2_anca)
  Constant4/1 -> Mux11/6
  [s_des] -> Mux10/1
  Demux6/2 -> Goto10/1
  [theta] -> Mux11/2
  Selector13/1 -> Demux8/1
  Selector14/1 -> Demux7/1
  Demux9/2 -> [q2]
  In4/1 -> [q3]
  [X] -> MATLAB Function9/1(X)
  Demux8/1 -> [s_dot_act]
  In5/1 -> [delta_s]
  MATLAB Function7/1(tau_leg) -> Demux6/1
  MATLAB Function8/2(theta) -> [theta]
  Constant7/1 -> Mux10/5
  [tau_w] -> Selector/1
  In6/1 -> [F_z]
  In2/1 -> Selector13/1
  From52/1 -> MATLAB Function7/2(q1_ginocchio)
  [theta_dot] -> Mux11/5
  [tau_k] -> Out2/1
  Demux9/1 -> [q1]
  MATLAB Function8/3(I_y) -> [Iy]
  [l_eq] -> MATLAB Function9/3(l)
  MATLAB Function8/4(theta_dot) -> [theta_dot]
  Demux6/1 -> Goto9/1
  Gain13/1 -> Mux10/2
  In1/1 -> Selector14/1
  Mux11/1 -> [X]
  [Iy] -> MATLAB Function9/4(I_y)
  [X_ref] -> MATLAB Function9/2(X_ref)
  MATLAB Function9/1(U) -> [tau_w]
  [s_dot_act] -> Mux11/4
  Constant/1 -> Mux11/3
  Mux10/1 -> [X_ref]
  Demux7/1 -> [s_act]
  MATLAB Function8/1(l) -> [l_eq]
  [q2] -> MATLAB Function8/2(q2_anca)
  [delta_s] -> Gain13/1
  [s_act] -> Mux11/1
  In3/1 -> Demux9/1
  Selector/1 -> Out3/1
  Constant1/1 -> Mux10/3
  Constant2/1 -> Mux10/6
  s_des/1 -> [s_des]
  s_dot_des/1 -> [s_dot_des]
  Step/1 -> MATLAB Function/1(Delta_s_des)
  [q1] -> MATLAB Function/3(q1_ginocchio)
  [q2] -> MATLAB Function/4(q2_anca)
  Demux1/1 -> [tau_k]
  Demux1/2 -> [tau_h]
  MATLAB Function/1(tau_leg) -> Demux1/1
  [F_z] -> MATLAB Function/2(F_z_mpc)

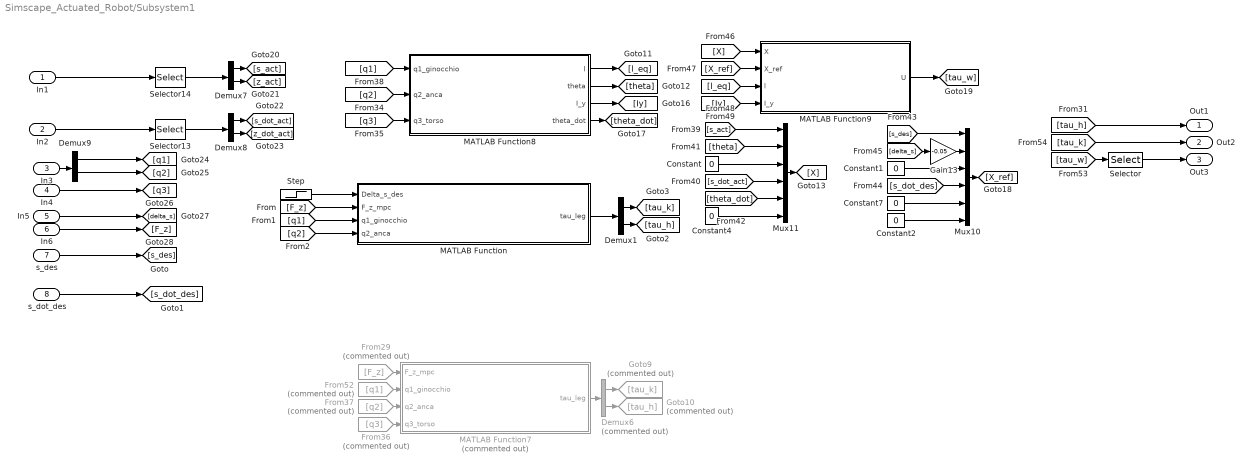
== system Simscape_Actuated_Robot/Subsystem1 ==
  In1 : Inport
  In2 : Inport  Port=2
  In3 : Inport  Port=3
  In4 : Inport  Port=4
  In5 : Inport  Port=5
  In6 : Inport  Port=6
  s_des : Inport  Port=7
  s_dot_des : Inport  Port=8
  Constant{,1..2,4,7} (5 alike) : Constant  Value=0
  Demux{1,7..9} (4 alike) : Demux  Outputs=2
  Demux6 : Demux  Commented=on  Outputs=2
  From29 : From  Commented=on  GotoTag=F_z
  From36 : From  Commented=on  GotoTag=q3
  From37 : From  Commented=on  GotoTag=q2
  From52 : From  Commented=on  GotoTag=q1
  Gain13 : Gain  Gain=-0.05
  Goto10 : Goto  Commented=on  GotoTag=tau_h
  Goto9 : Goto  Commented=on  GotoTag=tau_k
  MATLAB Function : MATLAB Function  TreatAsAtomicUnit=on
  MATLAB Function7 : MATLAB Function  Commented=on  TreatAsAtomicUnit=on
  MATLAB Function8 : MATLAB Function  TreatAsAtomicUnit=on
  MATLAB Function9 : MATLAB Function  TreatAsAtomicUnit=on
  Mux10 : Mux  Inputs=6
  Mux11 : Mux  Inputs=6
  Selector : Selector  InputPortWidth=2  IndexOptions=Index vector (dialog)  Indices=[1]  OutputSizes=1
  Selector13 : Selector  InputPortWidth=3  IndexOptions=Index vector (dialog)  Indices=[1 3]  OutputSizes=1
  Selector14 : Selector  InputPortWidth=3  IndexOptions=Index vector (dialog)  Indices=[1 3]  OutputSizes=1
  Step : Step  Time=2  After=0.05  SampleTime=Ts
  Out1 : Outport
  Out2 : Outport  Port=2
  Out3 : Outport  Port=3
  wires:
  Demux7/2 -> [z_act]
  From29/1 -> MATLAB Function7/1(F_z_mpc)
  [s_dot_des] -> Mux10/4
  [tau_h] -> Out1/1
  [q1] -> MATLAB Function8/1(q1_ginocchio)
  [q3] -> MATLAB Function8/3(q3_torso)
  From36/1 -> MATLAB Function7/4(q3_torso)
  Demux8/2 -> [z_dot_act]
  From37/1 -> MATLAB Function7/3(q2_anca)
  Constant4/1 -> Mux11/6
  [s_des] -> Mux10/1
  Demux6/2 -> Goto10/1
  [theta] -> Mux11/2
  Selector13/1 -> Demux8/1
  Selector14/1 -> Demux7/1
  Demux9/2 -> [q2]
  In4/1 -> [q3]
  [X] -> MATLAB Function9/1(X)
  Demux8/1 -> [s_dot_act]
  In5/1 -> [delta_s]
  MATLAB Function7/1(tau_leg) -> Demux6/1
  MATLAB Function8/2(theta) -> [theta]
  Constant7/1 -> Mux10/5
  [tau_w] -> Selector/1
  In6/1 -> [F_z]
  In2/1 -> Selector13/1
  From52/1 -> MATLAB Function7/2(q1_ginocchio)
  [theta_dot] -> Mux11/5
  [tau_k] -> Out2/1
  Demux9/1 -> [q1]
  MATLAB Function8/3(I_y) -> [Iy]
  [l_eq] -> MATLAB Function9/3(l)
  MATLAB Function8/4(theta_dot) -> [theta_dot]
  Demux6/1 -> Goto9/1
  Gain13/1 -> Mux10/2
  In1/1 -> Selector14/1
  Mux11/1 -> [X]
  [Iy] -> MATLAB Function9/4(I_y)
  [X_ref] -> MATLAB Function9/2(X_ref)
  MATLAB Function9/1(U) -> [tau_w]
  [s_dot_act] -> Mux11/4
  Constant/1 -> Mux11/3
  Mux10/1 -> [X_ref]
  Demux7/1 -> [s_act]
  MATLAB Function8/1(l) -> [l_eq]
  [q2] -> MATLAB Function8/2(q2_anca)
  [delta_s] -> Gain13/1
  [s_act] -> Mux11/1
  In3/1 -> Demux9/1
  Selector/1 -> Out3/1
  Constant1/1 -> Mux10/3
  Constant2/1 -> Mux10/6
  s_des/1 -> [s_des]
  s_dot_des/1 -> [s_dot_des]
  Step/1 -> MATLAB Function/1(Delta_s_des)
  [F_z] -> MATLAB Function/2(F_z_mpc)
  [q1] -> MATLAB Function/3(q1_ginocchio)
  [q2] -> MATLAB Function/4(q2_anca)
  Demux1/1 -> [tau_k]
  Demux1/2 -> [tau_h]
  MATLAB Function/1(tau_leg) -> Demux1/1

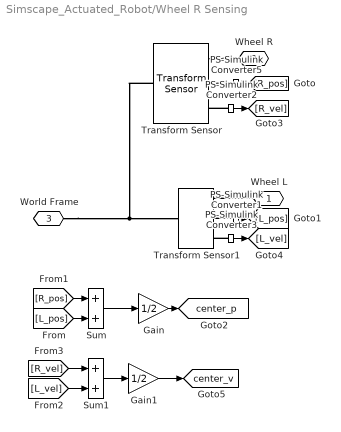
== system Simscape_Actuated_Robot/Wheel R Sensing ==
  Gain : Gain  Gain=1/2
  Gain1 : Gain  Gain=1/2
  PS-Simulink Converter{1..3,5} (4 alike) : nesl_utility/PS-Simulink Converter  PhysicalDomain=network_engine_domain  SubClassName=ps_output  LeftPortType=input  RightPortType=output  PseudoPeriodic=off  Frequencies=[]  VectorFormat=inherit  Unit=inherit  AffineConversion=off
  Sum : Sum
  Sum1 : Sum
  Transform Sensor : sm_lib/Frames and Transforms/Transform Sensor  MeasurementFrame=World  RotationSequence=XYZ  SenseAngle=off  SenseAxis=off  SenseQ=off  SenseR=off  SenseRotationSequence=off  SenseOmegaX=off  SenseOmegaY=off  SenseOmegaZ=off  SenseOmega=off  SenseQDot=off  SenseRDot=off  SenseRotationSequenceDot=off  SenseAlphaX=off  SenseAlphaY=off  SenseAlphaZ=off  SenseAlpha=off  SenseQDDot=off  SenseRDDot=off  SenseX=off  SenseY=off  SenseZ=off  SenseXYZ=on  SenseRad=off  SenseAzim=off  SenseDist=off  SenseInc=off  SenseXDot=off  SenseYDot=off  SenseZDot=off  SenseXYZDot=on  SenseRadDot=off  SenseAzimDot=off  SenseDistDot=off  SenseIncDot=off  SenseXDDot=off  SenseYDDot=off  SenseZDDot=off  SenseXYZDDot=off  SenseRadDDot=off  SenseAzimDDot=off  SenseDistDDot=off  SenseIncDDot=off
  Transform Sensor1 : sm_lib/Frames and Transforms/Transform Sensor  MeasurementFrame=World  RotationSequence=XYZ  SenseAngle=off  SenseAxis=off  SenseQ=off  SenseR=off  SenseRotationSequence=off  SenseOmegaX=off  SenseOmegaY=off  SenseOmegaZ=off  SenseOmega=off  SenseQDot=off  SenseRDot=off  SenseRotationSequenceDot=off  SenseAlphaX=off  SenseAlphaY=off  SenseAlphaZ=off  SenseAlpha=off  SenseQDDot=off  SenseRDDot=off  SenseX=off  SenseY=off  SenseZ=off  SenseXYZ=on  SenseRad=off  SenseAzim=off  SenseDist=off  SenseInc=off  SenseXDot=off  SenseYDot=off  SenseZDot=off  SenseXYZDot=on  SenseRadDot=off  SenseAzimDot=off  SenseDistDot=off  SenseIncDot=off  SenseXDDot=off  SenseYDDot=off  SenseZDDot=off  SenseXYZDDot=off  SenseRadDDot=off  SenseAzimDDot=off  SenseDistDDot=off  SenseIncDDot=off
  Wheel L : PMIOPort  Side=Left
  Wheel R : PMIOPort  Port=2  Side=Right
  "World Frame " : PMIOPort  Port=3  Side=Right
  tag scope: center_p=global, center_v=global
  wires:
  PS-Simulink Converter5/1 -> [R_pos]
  PS-Simulink Converter1/1 -> [L_pos]
  [R_pos] -> Sum/1
  [L_pos] -> Sum/2
  Sum/1 -> Gain/1
  Gain/1 -> [center_p]
  PS-Simulink Converter2/1 -> [R_vel]
  PS-Simulink Converter3/1 -> [L_vel]
  Sum1/1 -> Gain1/1
  [R_vel] -> Sum1/1
  [L_vel] -> Sum1/2
  Gain1/1 -> [center_v]
  connections:
  Transform Sensor/RConn1 -- Wheel R/RConn1
  "World Frame "/RConn1 -- Transform Sensor1/LConn1 -- Transform Sensor/LConn1
  PS-Simulink Converter5/LConn1 -- Transform Sensor/RConn2
  Wheel L/RConn1 -- Transform Sensor1/RConn1
  PS-Simulink Converter1/LConn1 -- Transform Sensor1/RConn2
  PS-Simulink Converter2/LConn1 -- Transform Sensor/RConn3
  PS-Simulink Converter3/LConn1 -- Transform Sensor1/RConn3

== matlab function Simscape_Actuated_Robot/MATLAB Function6 ==
  data: t input; s_des output; s_dot_des output
function [s_des, s_dot_des] = Smooth_Trajectory(t)
    % PRE-ALLOCAZIONE PER IL CODER
    s_des = 0.0;
    s_dot_des = 0.0;
    
    % PARAMETRI DELLA TRAIETTORIA
    t_start = 0.0;       % Il robot inizia a muoversi a 2 secondi
    t_end = 5.0;         % Arriva a destinazione a 5 secondi (3 secondi di viaggio)
    s_final = 1.0;       % Destinazione orizzontale (1 metro)
    
    % LOGICA DEL MOVIMENTO
    if t <= t_start
        % Prima di partire, resta fermo
        s_des = 0.0;
        s_dot_des = 0.0;
        
    elseif t >= t_end
        % Arrivato a destinazione, fermati
        s_des = s_final;
        s_dot_des = 0.0;
        
    else
        % FASE DI MOTO: Polinomio Cubico (Minimum Jerk Trajectory)
        % Normalizziamo il tempo tra 0 e 1 per la durata del viaggio
        tau = (t - t_start) / (t_end - t_start);
        
        % Posizione (Profilo a "S" morbida)
        s_des = s_final * (3*tau^2 - 2*tau^3);
        
        % Velocità (Derivata della posizione, forma a campana)
        s_dot_des = s_final * (6*tau - 6*tau^2) / (t_end - t_start);
    end
end

== matlab function Simscape_Actuated_Robot/Subsystem/MATLAB Function7 ==
  settings: updateMethod=DISCRETE
  data: tau_leg output; F_z_mpc input; q1_ginocchio input; q2_anca input; q3_torso input
function tau_leg  = VMC_Task_Space_Controller(F_z_mpc, q1_ginocchio, q2_anca, q3_torso)

% =========================================================================

% VMC CORRETTO - Ripartizione pulita delle competenze della GAMBA:

%   GINOCCHIO -> altezza z          (canale verticale)

%   ANCA      -> beccheggio torso q3 (stabilizzazione, anello prima mancante)

% Lo spostamento ORIZZONTALE del CoM NON e' piu' gestito qui: e' compito

% della ruota (TV-LQR). Cosi' sparisce il conflitto che destabilizzava l'MPC.

%

% Delta_s_des, s_actual, s_dot_actual, dq2_anca restano solo per compatibilita'

% di cablaggio (non sono piu' usati per il controllo dell'anca).

% =========================================================================
 
    % --- Uscite inizializzate (necessario per code generation) ---

    tau_leg   = zeros(2,1);

    SC_out    = 0.0;

    J_hip_out = 0.0;
 
    % --- Parametri fisici ---

    l1 = 0.45; l2 = 0.45;

    z_des = 0.6;          % altezza di equilibrio (asse ruota -> anca) [m]

    dt    = 0.001;        % deve coincidere col passo fisso del solutore
 
    % --- Stima derivate via differenza finita (persistenti) ---

    persistent q3_prev z_prev

    if isempty(q3_prev), q3_prev = q3_torso; end
 
    % Cinematica utile

    phi_shank = q1_ginocchio - q2_anca + q3_torso;

    phi_thigh = q3_torso - q2_anca;

    z_actual  = l1*cos(phi_shank) + l2*cos(phi_thigh);
 
    if isempty(z_prev), z_prev = z_actual; end
 
    dq3   = (q3_torso - q3_prev)/dt;   q3_prev = q3_torso;

    z_dot = (z_actual - z_prev)/dt;    z_prev  = z_actual;
 
    % --- CoM: solo per monitoraggio/uscite ---

    coder.extrinsic('calc_com_jacobian');

    J_SC = zeros(1,2); J_ZC = zeros(1,2); SC = 0.0; ZC = 0.0;

    [J_SC, J_ZC, SC, ZC] = calc_com_jacobian(q1_ginocchio, q2_anca, q3_torso);

    SC_out    = SC;

    J_hip_out = J_SC(2);
 
    % --- Compensazione di gravita' dalla dinamica VERA G(q) ---

    % (sostituisce il vecchio Jacobiano del ginocchio "clampato", instabile

    %  a gamba dritta). G non dipende da dq, quindi passo dq = 0.

    coder.extrinsic('calc_dynamics');

    q_full  = [q1_ginocchio; 0; q2_anca; q3_torso];   % ordine [q1;qw;q2;q3]

    M   = zeros(4,4); CdQ = zeros(4,1); G = zeros(4,1);

    [M, CdQ, G] = calc_dynamics(q_full, zeros(4,1));

    tau_k_grav = G(1);   % coppia statica ginocchio

    tau_h_grav = G(3);   % coppia statica anca
 
    % =====================================================================

    % (1) GINOCCHIO  ->  controllo di ALTEZZA

    % =====================================================================

    Kp_z = 4000; Kd_z = 300;               % PD altezza (DA TARARE)

    Jz_knee = -l1*sin(phi_shank);          % dz/dq1

    if abs(Jz_knee) < 0.05                  % vicino a gamba dritta: autorita' ~0

        Jz_knee = 0.05*sign(Jz_knee + 1e-9);

    end

    F_z_cmd = Kp_z*(z_des - z_actual) - Kd_z*z_dot + F_z_mpc;  % forza vert. extra

    tau_k   = tau_k_grav + Jz_knee * F_z_cmd;
 
    % =====================================================================

    % (2) ANCA  ->  stabilizza il BECCHEGGIO del torso  q3 -> 0

    % =====================================================================

    Kp_t = 800; Kd_t = 80;                 % PD torso (DA TARARE)

    % SEGNO: parti con -(Kp*q3 + Kd*dq3). Se in simulazione il torso DIVERGE

    %        invece di raddrizzarsi, INVERTI il segno del termine PD.

    tau_h = tau_h_grav - (Kp_t*q3_torso + Kd_t*dq3);
 
    tau_leg = [tau_k; tau_h];

end
